simulink model "Masking"  (R2024b)
settings: Solver=VariableStepAuto  StartTime=0.0  StopTime=10.0  RelTol=1e-3
settings Model: Creator=Ahmad  LastModifiedBy=Ahmad

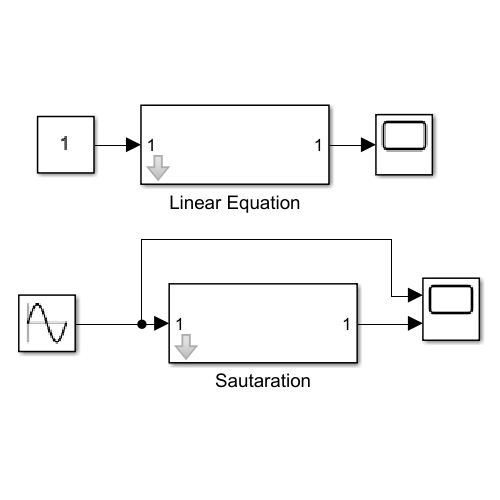
[thumbnail: Simulink's stored preview of the top-level diagram]
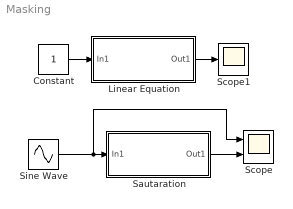
== system Masking ==
  Constant : Constant
  Linear Equation : Subsystem  mask{m=2, b=3}
      mask prompts: m "Slope"; b "Enter Section"
  Sautaration : Subsystem  mask{max_limit=0.5, min_limit=-0.5}
      mask prompts: max_limit "MAX"; min_limit "MIN"
  Scope : Scope  NumInputPorts=2
  Scope1 : Scope
  Sine Wave : Sin  SampleTime=0
  wires:
  Sine Wave/1 -> Scope/1, Sautaration/1(In1)
  Sautaration/1(Out1) -> Scope/2
  Constant/1 -> Linear Equation/1(In1)
  Linear Equation/1(Out1) -> Scope1/1

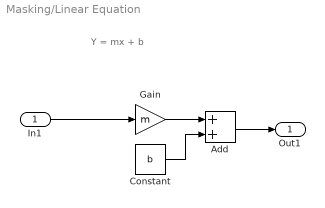
== system Masking/Linear Equation ==
  note: Y = mx + b
  In1 : Inport
  Add : Sum
  Constant : Constant  Value=b
  Gain : Gain  Gain=m
  Out1 : Outport
  wires:
  Add/1 -> Out1/1
  Gain/1 -> Add/1
  In1/1 -> Gain/1
  Constant/1 -> Add/2

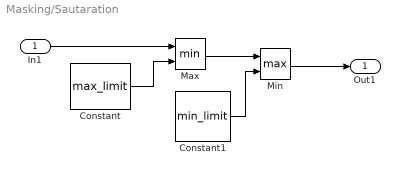
== system Masking/Sautaration ==
  In1 : Inport
  Constant : Constant  Value=max_limit
  Constant1 : Constant  Value=min_limit
  Max : MinMax  Inputs=2
  Min : MinMax  Function=max  Inputs=2
  Out1 : Outport
  wires:
  In1/1 -> Max/1
  Max/1 -> Min/1
  Constant/1 -> Max/2
  Constant1/1 -> Min/2
  Min/1 -> Out1/1
